simulink model "HighLevelMARCH"  (R2017a)
settings: Solver=FixedStepDiscrete  StartTime=0.0  StopTime=inf  FixedStep=0.002  RelTol=1e-3  EnableMultiTasking=on
undefined symbols (not defined in the file): DataLogger, ScopeHandler
libraries: slrtlib x8, LatchHandler x1, GESHandler x1, GaitHandler x1, InputDeviceHandler x1, JointHandler x1, OutCommunication x1, PowerElectronicsHandler x1, InCommunication x1, SOMANETHandler x1, StatemachineMARCH x1
settings Model: DataDictionary=ModelDictionary.sldd  SimulationMode=external  Creator=Taeke  LastModifiedBy=phil
settings SolverCC: EnableConcurrentExecution=on
settings DataIOCC: SaveFormat=StructureWithTime
settings OptimizationCC: BlockReduction=off  OptimizeBlockIOStorage=off  BufferReuse=off  GlobalBufferReuse=off  ExpressionFolding=off  LocalBlockOutputs=off
settings HardwareCC: ProdBitPerPointer=32  ProdBitPerSizeT=32  ProdBitPerPtrDiffT=32  ProdLargestAtomicFloat=None  ProdWordSize=32  ProdLongLongMode=on  ProdHWDeviceType=Generic->32-bit x86 compatible
settings RTWCC: SystemTargetFile=slrt.tlc  TemplateMakefile=slrt_default_tmf  Description=Simulink Real-Time  RTWCompilerOptimization=on
settings TargetCC: CodeReplacementLibrary=XPC_BLAS  ParMdlRefBuildCompliant=on  ConcurrentExecutionCompliant=on  GeneratePreprocessorConditionals=Use local settings  MatFileLogging=on  MATLABClassNameForMDSCustomization=xpcAperiodicCustomization

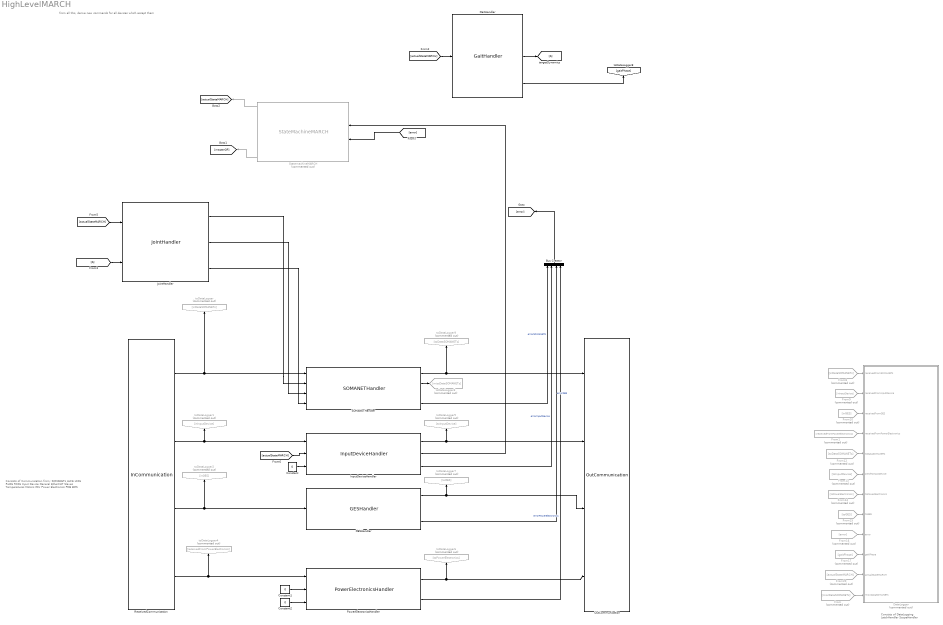
== system HighLevelMARCH ==
  note: from all this, derive new commands for all devices which accept them
  note: Consists of
      | DataLogging
      | LatchHandler
      | ScopeHandler
  note: Consists of Communication from:
      | SOMANETs
      | LHFE
      | LKFE
      | RHFE
      | RKFE
      | Input Device
      | General EtherCAT Slaves
      | Temperatures Motors
      | IMU
      | Power Electronics
      | PDB
      | BMS
  Bus Creator : BusCreator  Inputs=4  OutDataTypeStr=Bus: DeviceErrors  NonVirtualBus=on
  Constant : Constant  Value=0
  Constant1 : Constant  Value=0
  Constant2 : Constant  Value=0
  DataLogger : Subsystem  Commented=on  AncestorBlock=DataLogger/DataLogger
  From : From  Commented=on  GotoTag=miscDataSOMANETs
  From1 : From  Commented=on  GotoTag=receivedFromPowerElectronics
  From10 : From  Commented=on  GotoTag=inGES
  From12 : From  Commented=on  GotoTag=toDataSOMANETs
  From13 : From  Commented=on  GotoTag=toInputDevice
  From14 : From  Commented=on  GotoTag=toPowerElectronics
  From15 : From  Commented=on  GotoTag=toGES
  From16 : From  Commented=on  GotoTag=error
  From17 : From  Commented=on  GotoTag=gaitPhase
  From20 : From  Commented=on  GotoTag=actualStateMARCH
  From8 : From  Commented=on  GotoTag=inDataSOMANETs
  From9 : From  Commented=on  GotoTag=inInputDevice
  GESHandler : GESHandler/GESHandler
  GaitHandler : GaitHandler/GaitHandler
  InputDeviceHandler : InputDeviceHandler/InputDeviceHandler
  JointHandler : JointHandler/JointHandler
  OutCommunication : OutCommunication/OutCommunication
  PowerElectronicsHandler : PowerElectronicsHandler/PowerElectronicsHandler
  ReceivedCommunication : InCommunication/InCommunication
  SOMANETHandler : SOMANETHandler/SOMANETHandler
  StatemachineMARCH : StatemachineMARCH/StateMachineMARCH  Commented=on
  toDataLogger : Goto  Commented=on  GotoTag=inDataSOMANETs
  toDataLogger1 : Goto  Commented=on  GotoTag=inInputDevice
  toDataLogger2 : Goto  Commented=on  GotoTag=inGES
  toDataLogger3 : Goto  Commented=on  GotoTag=miscDataSOMANETs
  toDataLogger4 : Goto  Commented=on  GotoTag=receivedFromPowerElectronics
  toDataLogger5 : Goto  Commented=on  GotoTag=toInputDevice
  toDataLogger6 : Goto  Commented=on  GotoTag=toPowerElectronics
  toDataLogger7 : Goto  Commented=on  GotoTag=toGES
  toDataLogger9 : Goto  Commented=on  GotoTag=toDataSOMANETs
  wires:
  ReceivedCommunication/4 -> PowerElectronicsHandler/1, toDataLogger4/1
  ReceivedCommunication/3 -> GESHandler/1, toDataLogger2/1
  ReceivedCommunication/2 -> InputDeviceHandler/1, toDataLogger1/1
  ReceivedCommunication/1 -> SOMANETHandler/1, toDataLogger/1
  [actualStateMARCH] -> InputDeviceHandler/2
  [actualStateMARCH] -> JointHandler/1
  InputDeviceHandler/2 -> StatemachineMARCH/2
  [error] -> StatemachineMARCH/3
  SOMANETHandler/1 -> OutCommunication/1, toDataLogger9/1
  InputDeviceHandler/1 -> OutCommunication/2, toDataLogger5/1
  GESHandler/1 -> OutCommunication/3, toDataLogger7/1
  PowerElectronicsHandler/1 -> OutCommunication/4, toDataLogger6/1
  From8/1 -> DataLogger/1(receivedFromSOMANETs)
  From20/1 -> DataLogger/11(actualStateMARCH)
  From16/1 -> DataLogger/9(error)
  From9/1 -> DataLogger/2(receivedFromInputDevice)
  From10/1 -> DataLogger/3(receivedFromGES)
  From14/1 -> DataLogger/7(toPowerElectronics)
  From15/1 -> DataLogger/8(toGES)
  From17/1 -> DataLogger/10(gaitPhase)
  From1/1 -> DataLogger/4(receivedFromPowerElectronics)
  From12/1 -> DataLogger/5(toDataSOMANETs)
  From13/1 -> DataLogger/6(sendToInputDevice)
  From/1 -> DataLogger/12(miscDataSOMANETs)
  StatemachineMARCH/1 -> [actualStateMARCH]
  StatemachineMARCH/6 -> [masterOP]
  SOMANETHandler/2 -> toDataLogger3/1
  Bus Creator/1 -> [error]
  Constant/1 -> InputDeviceHandler/3
  SOMANETHandler/4 -> Bus Creator/1  "errorSOMANETs"
  InputDeviceHandler/3 -> Bus Creator/2  "errorInputDevice"
  GESHandler/3 -> Bus Creator/3  "errorGES"
  PowerElectronicsHandler/2 -> Bus Creator/4  "errorPowerElectronics"
  Constant1/1 -> PowerElectronicsHandler/2
  Constant2/1 -> PowerElectronicsHandler/3
  GaitHandler/3 -> [gaitPhase]
  [actualStateMARCH] -> GaitHandler/1
  JointHandler/1 -> SOMANETHandler/2
  JointHandler/2 -> SOMANETHandler/3
  GaitHandler/2 -> [A]
  [A] -> JointHandler/2
  JointHandler/3 -> SOMANETHandler/4

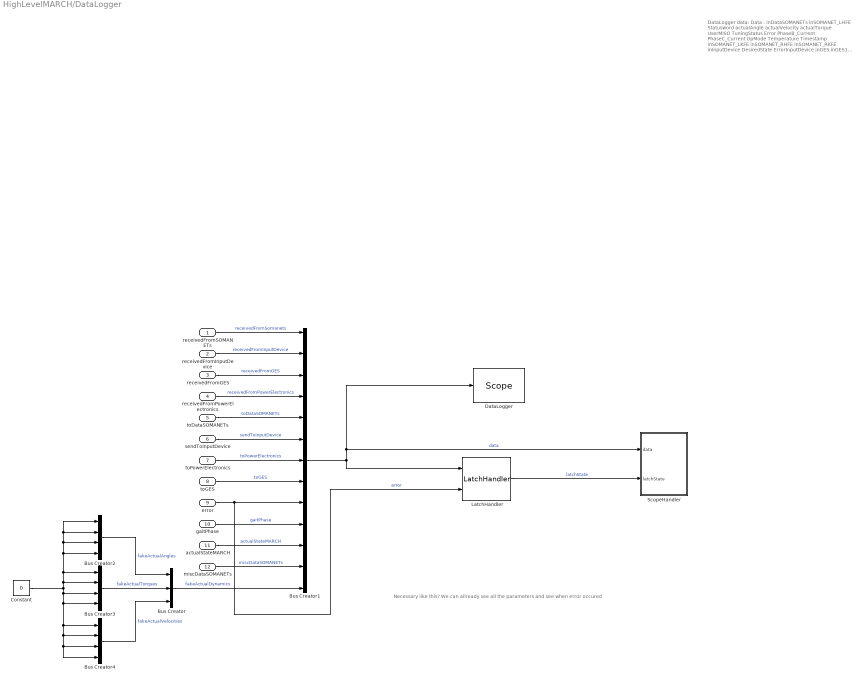
== system HighLevelMARCH/DataLogger ==
  note: Necessary like this? We can allready see all the parameters and see when error occured
  note: DataLogger data:
      | Data :
      | inDataSOMANETs
      | inSOMANET_LHFE
      | Statusword
      | actualAngle
      | actualVelocity
      | actualTorque
      | UserMISO
      | TuningStatus
      | Error
      | PhaseB_Current
      | PhaseC_Current
      | OpMode
      | Temperature
      | Timestamp
      | inSOMANET_LKFE
      | inSOMANET_RHFE
      | inSOMANET_RKFE
      | inInputDevice
      | DesiredState
      | ErrorInputDevice
      | inGES
      | inGES1
      | TempMotor
      | inGES2
      | inGES3
      | inGES4
      | inPowerElectronics
      | statusPDB
      | statusBMS
      | toDataSOMANETs
      | toSOMANET_LHFE
      | Controlword
      | OpMode
      | targetAngle
      | targetVelocity
      | targetTorque
      | TuningCommand
      | UserMOSI
      | maxTorque
      | toSOMANET_LKFE
      | toSOMANET_RHFE
      | toSOMANET_RKFE
      | toInputDevice
      | actualStateMARCH
      | Error
      | toPowerElectronics
      | toPDB
      | MasterOP
      | toGES
      | -
      | Error
      | ErrorSOMANETs
      | ErrorSOMANET_LHFE
      | ErrorSOMANET_LKFE
      | ErrorSOMANET_RHFE
      | ErrorSOMANET_RKFE
      | ErrorInputDevice
      | ErrorGES
      | ErrorGES1
      | ErrorGES2
      | ErrorGES3
      | ErrorGES4
      | ErrorPowerElectronics
      | ErrorPDB
      | ErrorBMS
      | GaitPhase
      | actualStateMARCH
      | ConfigSOMANETs
      | AngleOffset
      | PolePairs
      | minPosLimit
      | maxPosLimit
      | maxSpeed
      | maxTorque
      | PositionKp
      | PositionKi
      | PositionKd
      | PositionIntegralLimit
      | VelocityKp
      | VelocityKi
      | VelocityKd
      | VelocityIntegralLimit
      | BreakReleaseStrategy
      | calculatedDynamics
      | LatchState :
      | All data on specific error moment
  receivedFromSOMANETs : Inport  OutDataTypeStr=Bus: EtherCATReceivedFromSOMANET  PortDimensions=[1 4]  LockScale=on  BusOutputAsStruct=on
  receivedFromInputDevice : Inport  Port=2  OutDataTypeStr=Bus: EtherCATReceivedFromInputDevice  BusOutputAsStruct=on
  receivedFromGES : Inport  Port=3  OutDataTypeStr=Bus: EtherCATReceivedFromGES  BusOutputAsStruct=on
  receivedFromPowerElectronics : Inport  Port=4  OutDataTypeStr=Bus: EtherCATReceivedFromPowerElectronics  BusOutputAsStruct=on
  toDataSOMANETs : Inport  Port=5  OutDataTypeStr=Bus: toDataSOMANETs  BusOutputAsStruct=on
  sendToInputDevice : Inport  Port=6  OutDataTypeStr=Bus: EtherCATSendToInputDevice  BusOutputAsStruct=on
  toPowerElectronics : Inport  Port=7  OutDataTypeStr=Bus: toPowerElectronics  BusOutputAsStruct=on
  toGES : Inport  Port=8  OutDataTypeStr=Bus: toGES  BusOutputAsStruct=on
  error : Inport  Port=9  OutDataTypeStr=Bus: error  BusOutputAsStruct=on
  gaitPhase : Inport  Port=10
  actualStateMARCH : Inport  Port=11
  miscDataSOMANETs : Inport  Port=12  OutDataTypeStr=Bus: MiscDataSOMANET  BusOutputAsStruct=on
  Bus Creator : BusCreator  Inputs=3  OutDataTypeStr=Bus: calculatedDynamics
  Bus Creator1 : BusCreator  Inputs=13  OutDataTypeStr=Bus: ExoskeletonData  NonVirtualBus=on
  Bus Creator2 : BusCreator  Inputs=4  OutDataTypeStr=Bus: calculatedAngles
  Bus Creator3 : BusCreator  Inputs=4  OutDataTypeStr=Bus: calculatedTorques
  Bus Creator4 : BusCreator  Inputs=4  OutDataTypeStr=Bus: calculatedVelocities
  Constant : Constant  Value=0
  "DataLogger " : slrtlib/Displays and Logging/Scope   scopeno=10  scopetype=File  autostart=on  viewmode=Graphical redraw  formatstr='%15.6f'  grid=on  ylimits=[0,0]  nosamples=4600000  noprepostsamples=0  interleave=1  triggermode=FreeRun  triggersignal=1  trigsignalfromport=off  triggerlevel=0.0  triggerslope=Either  triggerscope=1  triggersample=0  filename=MARCH.dat  mode=Lazy  writesize=512  autorestart=off  dynamicfilemode=off  maxwritefilesize=512*1024^2
  LatchHandler : LatchHandler/LatchHandler
  ScopeHandler : Subsystem  AncestorBlock=ScopeHandler/ScopeHandler
  wires:
  error/1 -> Bus Creator1/9, LatchHandler/2  "error"
  Bus Creator1/1 -> "DataLogger "/1, ScopeHandler/1(data), LatchHandler/1  "data"
  LatchHandler/1 -> ScopeHandler/2(latchState)  "latchState"
  Constant/1 -> Bus Creator3/3, Bus Creator3/4, Bus Creator4/1, Bus Creator4/2, Bus Creator4/3, Bus Creator4/4, Bus Creator3/2, Bus Creator3/1, Bus Creator2/4, Bus Creator2/3, Bus Creator2/2, Bus Creator2/1
  Bus Creator3/1 -> Bus Creator/2  "fakeActualTorques"
  Bus Creator2/1 -> Bus Creator/1  "fakeActualAngles"
  Bus Creator4/1 -> Bus Creator/3  "fakeActualVelocities"
  receivedFromSOMANETs/1 -> Bus Creator1/1  "receivedFromSomanets"
  receivedFromInputDevice/1 -> Bus Creator1/2  "receivedFromInputDevice"
  receivedFromGES/1 -> Bus Creator1/3  "receivedFromGES"
  receivedFromPowerElectronics/1 -> Bus Creator1/4  "receivedFromPowerElectronics"
  toDataSOMANETs/1 -> Bus Creator1/5  "toDataSOMANETs"
  sendToInputDevice/1 -> Bus Creator1/6  "sendToInputDevice"
  toPowerElectronics/1 -> Bus Creator1/7  "toPowerElectronics"
  toGES/1 -> Bus Creator1/8  "toGES"
  gaitPhase/1 -> Bus Creator1/10  "gaitPhase"
  actualStateMARCH/1 -> Bus Creator1/11  "actualStateMARCH"
  miscDataSOMANETs/1 -> Bus Creator1/12  "miscDataSOMANETs"
  Bus Creator/1 -> Bus Creator1/13  "fakeActualDynamics"

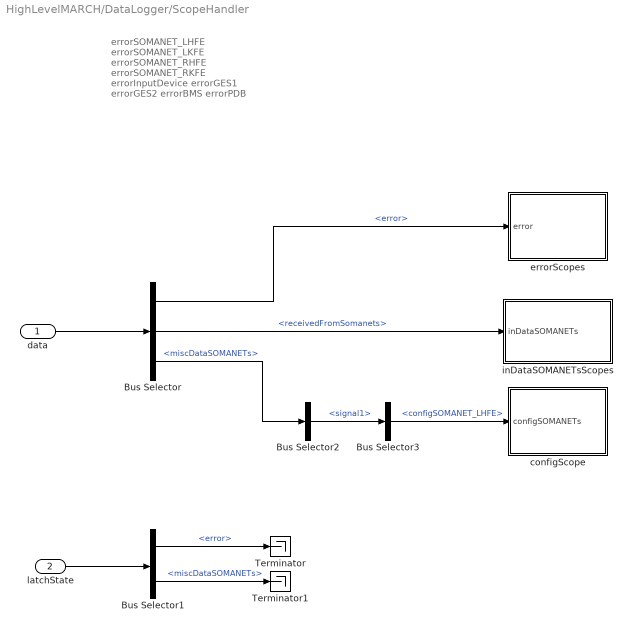
== system HighLevelMARCH/DataLogger/ScopeHandler ==
  note: errorSOMANET_LHFE
      | errorSOMANET_LKFE
      | errorSOMANET_RHFE
      | errorSOMANET_RKFE
      | errorInputDevice
      | errorGES1
      | errorGES2
      | errorBMS
      | errorPDB
  data : Inport  OutDataTypeStr=Bus: ExoskeletonData  BusOutputAsStruct=on
  latchState : Inport  Port=2  OutDataTypeStr=Bus: ExoskeletonData  BusOutputAsStruct=on
  Bus Selector : BusSelector  OutputSignals=error,receivedFromSomanets,miscDataSOMANETs
  Bus Selector1 : BusSelector  OutputSignals=error,miscDataSOMANETs
  Bus Selector2 : BusSelector  OutputSignals=signal1
  Bus Selector3 : BusSelector  OutputSignals=configSOMANET_LHFE
  Terminator : Terminator
  Terminator1 : Terminator
  configScope : Subsystem
  errorScopes : Subsystem
  inDataSOMANETsScopes : Subsystem
  wires:
  latchState/1 -> Bus Selector1/1
  data/1 -> Bus Selector/1
  Bus Selector/1 -> errorScopes/1(error)  "<error>"
  Bus Selector/2 -> inDataSOMANETsScopes/1(inDataSOMANETs)  "<receivedFromSomanets>"
  Bus Selector1/1 -> Terminator/1  "<error>"
  Bus Selector1/2 -> Terminator1/1  "<miscDataSOMANETs>"
  Bus Selector/3 -> Bus Selector2/1  "<miscDataSOMANETs>"
  Bus Selector2/1 -> Bus Selector3/1  "<signal1>"
  Bus Selector3/1 -> configScope/1(configSOMANETs)  "<configSOMANET_LHFE>"

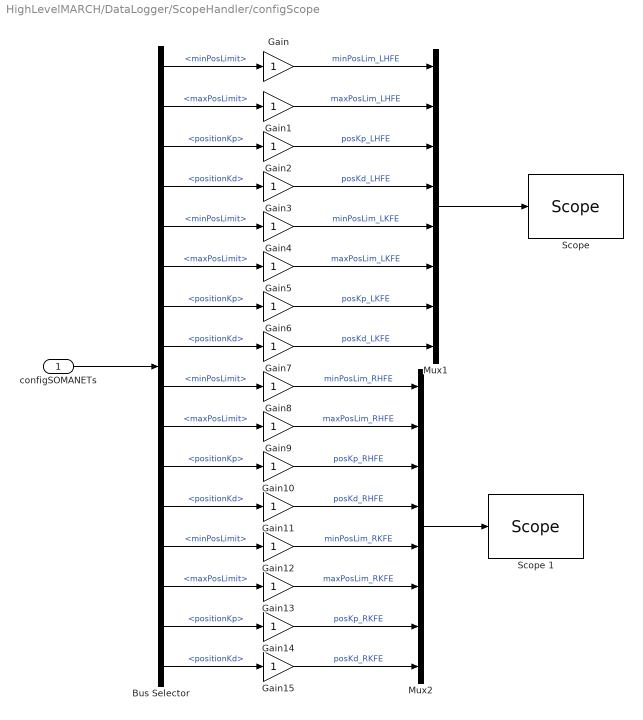
== system HighLevelMARCH/DataLogger/ScopeHandler/configScope ==
  configSOMANETs : Inport
  Bus Selector : BusSelector  OutputSignals=minPosLimit,maxPosLimit,positionKp,positionKd,minPosLimit,maxPosLimit,positionKp,positionKd,minPosLimit,maxPosLimit,positionKp,positionKd,minPosLimit,maxPosLimit,positionKp,positionKd
  Gain{,1..15} (16 alike) : Gain
  Mux1 : Mux  Inputs=8
  Mux2 : Mux  Inputs=8
  "Scope " : slrtlib/Displays and Logging/Scope   scopeno=6  scopetype=Target  autostart=on  viewmode=Numerical  formatstr='%15.6f'  grid=on  ylimits=[0,0]  nosamples=250  noprepostsamples=0  interleave=1  triggermode=FreeRun  triggersignal=1  trigsignalfromport=off  triggerlevel=0.0  triggerslope=Either  triggerscope=1  triggersample=0  filename=data.dat  mode=Lazy  writesize=512  autorestart=off  dynamicfilemode=off  maxwritefilesize=512*1024^2
  Scope 1 : slrtlib/Displays and Logging/Scope   scopeno=7  scopetype=Target  autostart=on  viewmode=Numerical  formatstr='%15.6f'  grid=on  ylimits=[0,0]  nosamples=250  noprepostsamples=0  interleave=1  triggermode=FreeRun  triggersignal=1  trigsignalfromport=off  triggerlevel=0.0  triggerslope=Either  triggerscope=1  triggersample=0  filename=data.dat  mode=Lazy  writesize=512  autorestart=off  dynamicfilemode=off  maxwritefilesize=512*1024^2
  wires:
  configSOMANETs/1 -> Bus Selector/1
  Bus Selector/4 -> Gain3/1  "<positionKd>"
  Bus Selector/5 -> Gain4/1  "<minPosLimit>"
  Bus Selector/6 -> Gain5/1  "<maxPosLimit>"
  Bus Selector/7 -> Gain6/1  "<positionKp>"
  Bus Selector/8 -> Gain7/1  "<positionKd>"
  Bus Selector/9 -> Gain8/1  "<minPosLimit>"
  Bus Selector/10 -> Gain9/1  "<maxPosLimit>"
  Bus Selector/11 -> Gain10/1  "<positionKp>"
  Bus Selector/12 -> Gain11/1  "<positionKd>"
  Bus Selector/13 -> Gain12/1  "<minPosLimit>"
  Bus Selector/14 -> Gain13/1  "<maxPosLimit>"
  Bus Selector/15 -> Gain14/1  "<positionKp>"
  Bus Selector/16 -> Gain15/1  "<positionKd>"
  Mux2/1 -> Scope 1/1
  Mux1/1 -> "Scope "/1
  Gain/1 -> Mux1/1  "minPosLim_LHFE"
  Gain1/1 -> Mux1/2  "maxPosLim_LHFE"
  Gain2/1 -> Mux1/3  "posKp_LHFE"
  Gain3/1 -> Mux1/4  "posKd_LHFE"
  Gain4/1 -> Mux1/5  "minPosLim_LKFE"
  Gain5/1 -> Mux1/6  "maxPosLim_LKFE"
  Gain6/1 -> Mux1/7  "posKp_LKFE"
  Gain7/1 -> Mux1/8  "posKd_LKFE"
  Gain8/1 -> Mux2/1  "minPosLim_RHFE"
  Gain9/1 -> Mux2/2  "maxPosLim_RHFE"
  Gain10/1 -> Mux2/3  "posKp_RHFE"
  Gain11/1 -> Mux2/4  "posKd_RHFE"
  Gain12/1 -> Mux2/5  "minPosLim_RKFE"
  Gain13/1 -> Mux2/6  "maxPosLim_RKFE"
  Gain14/1 -> Mux2/7  "posKp_RKFE"
  Gain15/1 -> Mux2/8  "posKd_RKFE"
  Bus Selector/3 -> Gain2/1  "<positionKp>"
  Bus Selector/2 -> Gain1/1  "<maxPosLimit>"
  Bus Selector/1 -> Gain/1  "<minPosLimit>"

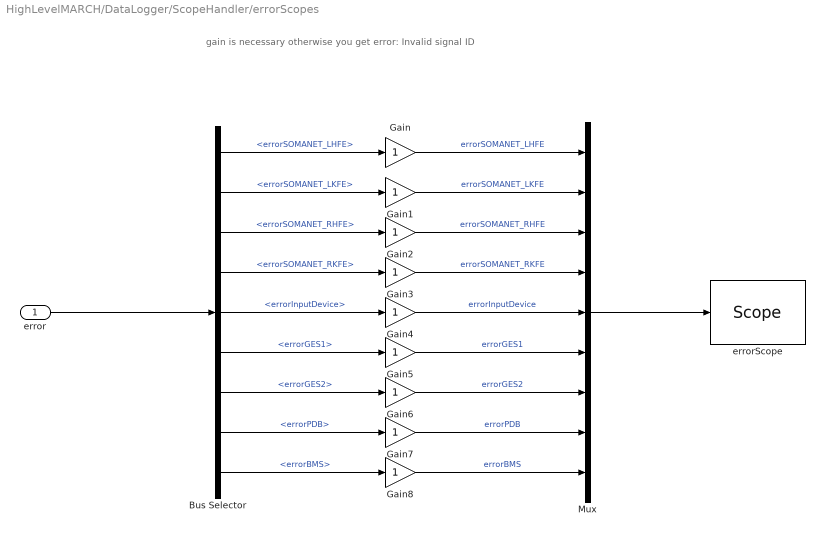
== system HighLevelMARCH/DataLogger/ScopeHandler/errorScopes ==
  note: gain is necessary otherwise you get error: Invalid signal ID
  error : Inport
  Bus Selector : BusSelector  OutputSignals=signal1.errorSOMANET_LHFE,signal1.errorSOMANET_LKFE,signal1.errorSOMANET_RHFE,signal1.errorSOMANET_RKFE,errorInputDevice,signal3.errorGES1,signal3.errorGES2,signal4.errorPDB,signal4.errorBMS
  Gain{,1..8} (9 alike) : Gain
  Mux : Mux  Inputs=9
  errorScope : slrtlib/Displays and Logging/Scope   scopeno=5  scopetype=Target  autostart=on  viewmode=Numerical  formatstr='%15.6f'  grid=on  ylimits=[0,0]  nosamples=250  noprepostsamples=0  interleave=1  triggermode=FreeRun  triggersignal=1  trigsignalfromport=off  triggerlevel=0.0  triggerslope=Either  triggerscope=1  triggersample=0  filename=data.dat  mode=Lazy  writesize=512  autorestart=off  dynamicfilemode=off  maxwritefilesize=512*1024^2
  wires:
  error/1 -> Bus Selector/1
  Bus Selector/1 -> Gain/1  "<errorSOMANET_LHFE>"
  Bus Selector/2 -> Gain1/1  "<errorSOMANET_LKFE>"
  Bus Selector/3 -> Gain2/1  "<errorSOMANET_RHFE>"
  Bus Selector/4 -> Gain3/1  "<errorSOMANET_RKFE>"
  Bus Selector/5 -> Gain4/1  "<errorInputDevice>"
  Bus Selector/6 -> Gain5/1  "<errorGES1>"
  Bus Selector/7 -> Gain6/1  "<errorGES2>"
  Bus Selector/8 -> Gain7/1  "<errorPDB>"
  Bus Selector/9 -> Gain8/1  "<errorBMS>"
  Mux/1 -> errorScope/1
  Gain/1 -> Mux/1  "errorSOMANET_LHFE"
  Gain1/1 -> Mux/2  "errorSOMANET_LKFE"
  Gain2/1 -> Mux/3  "errorSOMANET_RHFE"
  Gain3/1 -> Mux/4  "errorSOMANET_RKFE"
  Gain4/1 -> Mux/5  "errorInputDevice"
  Gain5/1 -> Mux/6  "errorGES1"
  Gain6/1 -> Mux/7  "errorGES2"
  Gain7/1 -> Mux/8  "errorPDB"
  Gain8/1 -> Mux/9  "errorBMS"

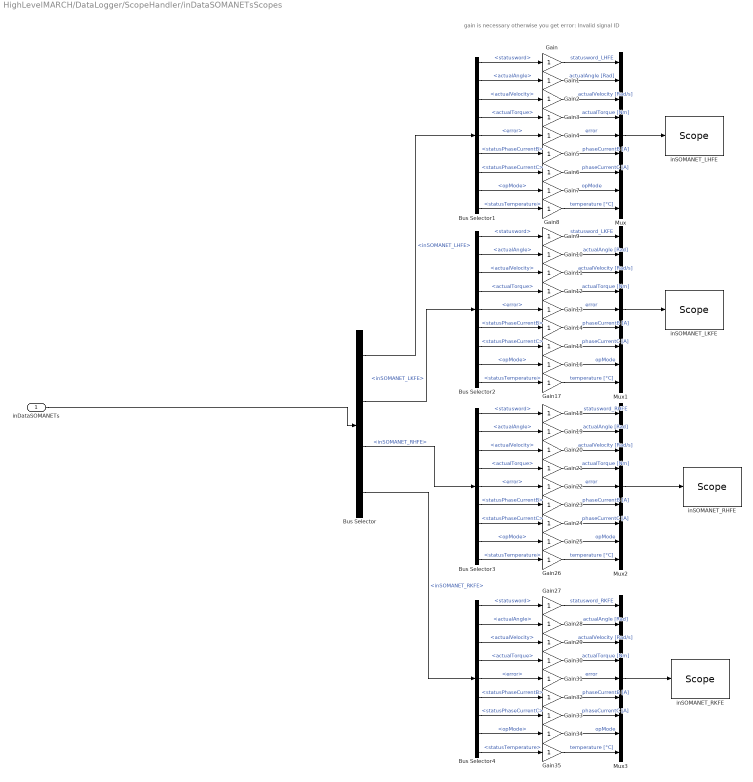
== system HighLevelMARCH/DataLogger/ScopeHandler/inDataSOMANETsScopes ==
  note: gain is necessary otherwise you get error: Invalid signal ID
  inDataSOMANETs : Inport
  Bus Selector : BusSelector  OutputSignals=inSOMANET_LHFE,inSOMANET_LKFE,inSOMANET_RHFE,inSOMANET_RKFE
  Bus Selector{1..4} (4 alike) : BusSelector  OutputSignals=statusword,actualAngle,actualVelocity,actualTorque,error,statusPhaseCurrentB,statusPhaseCurrentC,opMode,statusTemperature
  Gain{,1..35} (36 alike) : Gain
  Mux{,1..3} (4 alike) : Mux  Inputs=9
  inSOMANET_LHFE : slrtlib/Displays and Logging/Scope   scopeno=1  scopetype=Target  autostart=on  viewmode=Numerical  formatstr='%15.6f'  grid=on  ylimits=[0,0]  nosamples=250  noprepostsamples=0  interleave=1  triggermode=FreeRun  triggersignal=1  trigsignalfromport=off  triggerlevel=0.0  triggerslope=Either  triggerscope=1  triggersample=0  filename=data.dat  mode=Lazy  writesize=512  autorestart=off  dynamicfilemode=off  maxwritefilesize=512*1024^2
  "inSOMANET_LKFE " : slrtlib/Displays and Logging/Scope   scopeno=2  scopetype=Target  autostart=on  viewmode=Numerical  formatstr='%15.6f'  grid=on  ylimits=[0,0]  nosamples=250  noprepostsamples=0  interleave=1  triggermode=FreeRun  triggersignal=1  trigsignalfromport=off  triggerlevel=0.0  triggerslope=Either  triggerscope=1  triggersample=0  filename=data.dat  mode=Lazy  writesize=512  autorestart=off  dynamicfilemode=off  maxwritefilesize=512*1024^2
  inSOMANET_RHFE : slrtlib/Displays and Logging/Scope   scopeno=3  scopetype=Target  autostart=on  viewmode=Numerical  formatstr='%15.6f'  grid=on  ylimits=[0,0]  nosamples=250  noprepostsamples=0  interleave=1  triggermode=FreeRun  triggersignal=1  trigsignalfromport=off  triggerlevel=0.0  triggerslope=Either  triggerscope=1  triggersample=0  filename=data.dat  mode=Lazy  writesize=512  autorestart=off  dynamicfilemode=off  maxwritefilesize=512*1024^2
  inSOMANET_RKFE : slrtlib/Displays and Logging/Scope   scopeno=4  scopetype=Target  autostart=on  viewmode=Numerical  formatstr='%15.6f'  grid=on  ylimits=[0,0]  nosamples=250  noprepostsamples=0  interleave=1  triggermode=FreeRun  triggersignal=1  trigsignalfromport=off  triggerlevel=0.0  triggerslope=Either  triggerscope=1  triggersample=0  filename=data.dat  mode=Lazy  writesize=512  autorestart=off  dynamicfilemode=off  maxwritefilesize=512*1024^2
  wires:
  inDataSOMANETs/1 -> Bus Selector/1
  Bus Selector/1 -> Bus Selector1/1  "<inSOMANET_LHFE>"
  Bus Selector/2 -> Bus Selector2/1  "<inSOMANET_LKFE>"
  Bus Selector/3 -> Bus Selector3/1  "<inSOMANET_RHFE>"
  Bus Selector/4 -> Bus Selector4/1  "<inSOMANET_RKFE>"
  Bus Selector1/1 -> Gain/1  "<statusword>"
  Bus Selector1/2 -> Gain1/1  "<actualAngle>"
  Bus Selector1/3 -> Gain2/1  "<actualVelocity>"
  Bus Selector1/4 -> Gain3/1  "<actualTorque>"
  Bus Selector1/5 -> Gain4/1  "<error>"
  Bus Selector1/6 -> Gain5/1  "<statusPhaseCurrentB>"
  Bus Selector1/7 -> Gain6/1  "<statusPhaseCurrentC>"
  Bus Selector2/1 -> Gain9/1  "<statusword>"
  Bus Selector2/2 -> Gain10/1  "<actualAngle>"
  Bus Selector2/3 -> Gain11/1  "<actualVelocity>"
  Bus Selector2/4 -> Gain12/1  "<actualTorque>"
  Bus Selector2/5 -> Gain13/1  "<error>"
  Bus Selector2/6 -> Gain14/1  "<statusPhaseCurrentB>"
  Bus Selector2/7 -> Gain15/1  "<statusPhaseCurrentC>"
  Bus Selector3/1 -> Gain18/1  "<statusword>"
  Bus Selector3/2 -> Gain19/1  "<actualAngle>"
  Bus Selector3/3 -> Gain20/1  "<actualVelocity>"
  Bus Selector3/4 -> Gain21/1  "<actualTorque>"
  Bus Selector3/5 -> Gain22/1  "<error>"
  Bus Selector3/6 -> Gain23/1  "<statusPhaseCurrentB>"
  Bus Selector3/7 -> Gain24/1  "<statusPhaseCurrentC>"
  Bus Selector4/1 -> Gain27/1  "<statusword>"
  Bus Selector4/2 -> Gain28/1  "<actualAngle>"
  Bus Selector4/3 -> Gain29/1  "<actualVelocity>"
  Bus Selector4/4 -> Gain30/1  "<actualTorque>"
  Bus Selector4/5 -> Gain31/1  "<error>"
  Bus Selector4/6 -> Gain32/1  "<statusPhaseCurrentB>"
  Bus Selector4/7 -> Gain33/1  "<statusPhaseCurrentC>"
  Bus Selector4/8 -> Gain34/1  "<opMode>"
  Bus Selector4/9 -> Gain35/1  "<statusTemperature>"
  Bus Selector3/8 -> Gain25/1  "<opMode>"
  Bus Selector3/9 -> Gain26/1  "<statusTemperature>"
  Bus Selector2/8 -> Gain16/1  "<opMode>"
  Bus Selector2/9 -> Gain17/1  "<statusTemperature>"
  Bus Selector1/8 -> Gain7/1  "<opMode>"
  Bus Selector1/9 -> Gain8/1  "<statusTemperature>"
  Mux3/1 -> inSOMANET_RKFE/1
  Mux2/1 -> inSOMANET_RHFE/1
  Mux1/1 -> "inSOMANET_LKFE "/1
  Mux/1 -> inSOMANET_LHFE/1
  Gain/1 -> Mux/1  "statusword_LHFE"
  Gain1/1 -> Mux/2  "actualAngle [Rad]"
  Gain2/1 -> Mux/3  "actualVelocity [Rad/s]"
  Gain3/1 -> Mux/4  "actualTorque [Nm]"
  Gain4/1 -> Mux/5  "error"
  Gain5/1 -> Mux/6  "phaseCurrentB [A]"
  Gain6/1 -> Mux/7  "phaseCurrentC [A]"
  Gain7/1 -> Mux/8  "opMode"
  Gain8/1 -> Mux/9  "temperature [°C]"
  Gain9/1 -> Mux1/1  "statusword_LKFE"
  Gain14/1 -> Mux1/6  "phaseCurrentB [A]"
  Gain15/1 -> Mux1/7  "phaseCurrentC [A]"
  Gain11/1 -> Mux1/3  "actualVelocity [Rad/s]"
  Gain13/1 -> Mux1/5  "error"
  Gain12/1 -> Mux1/4  "actualTorque [Nm]"
  Gain10/1 -> Mux1/2  "actualAngle [Rad]"
  Gain17/1 -> Mux1/9  "temperature [°C]"
  Gain16/1 -> Mux1/8  "opMode"
  Gain18/1 -> Mux2/1  "statusword_RHFE"
  Gain21/1 -> Mux2/4  "actualTorque [Nm]"
  Gain19/1 -> Mux2/2  "actualAngle [Rad]"
  Gain20/1 -> Mux2/3  "actualVelocity [Rad/s]"
  Gain26/1 -> Mux2/9  "temperature [°C]"
  Gain23/1 -> Mux2/6  "phaseCurrentB [A]"
  Gain25/1 -> Mux2/8  "opMode"
  Gain24/1 -> Mux2/7  "phaseCurrentC [A]"
  Gain22/1 -> Mux2/5  "error"
  Gain30/1 -> Mux3/4  "actualTorque [Nm]"
  Gain33/1 -> Mux3/7  "phaseCurrentC [A]"
  Gain31/1 -> Mux3/5  "error"
  Gain32/1 -> Mux3/6  "phaseCurrentB [A]"
  Gain34/1 -> Mux3/8  "opMode"
  Gain35/1 -> Mux3/9  "temperature [°C]"
  Gain27/1 -> Mux3/1  "statusword_RKFE"
  Gain29/1 -> Mux3/3  "actualVelocity [Rad/s]"
  Gain28/1 -> Mux3/2  "actualAngle [Rad]"
